simulink model "different_inverter_controls_BPS"  (R2024b)
settings: Solver=ode4  StartTime=0.0  StopTime=5  FixedStep=Ts  RelTol=1e-3
InitFcn:
  | %mode_of_operation=1;
  | %BESS_control_mode=1;
  | %Gen_Q_Control =1;
  | 
  | %Exciter_init;
  | 
  | %Exciter_init
  | Xq=0.474;
  | %%====================================================
  | % ST6C Exciter Parameters
  | 
  | KPA=30;
  | KIA=59.91;
  | KFF=1;
  | KM=1;
  | KLR=22.47;
  | KCL=1.04;
  | VAMAX=7.05;
  | VAMIN=-6.11;
  | VRMAX=7.05;
  | VRMIN=-6.11;
  | ILR=5.02;
  | KG=1;
  | TG=0.024;
  | TA=0.01;
  | VBMAX=999;
  | VMMAX=7.05;
  | VMMIN=-6.11;
  | KI=0;
  | Kp=1;
  | Kc=0;
  | Vt0=0;
  | VAAMAX=VAMAX;
  | %%========================================================
  | % UEL2C parameters
  | 
  | TUQ=.005;
  | TUP=0.050;
  | TUV=0.2;
  | TQREF=0;
  | Tadj=0;
  | K1=0;
  | K2=2;
  | VBIAS=1;
  | KFB=0;
  | TUL=0;
  | VUImax=1;
  | VUImin=-1;
  | VUELmax1=1;
  | VUELmax2=1;
  | VUELmin1=-1;
  | VUELmin2=-1;
  | KUF=0;
  | KUL=0.24;
  | KUI=0.001;
  | TU1=0;TU2=0;TU3=0;TU4=0;
  | KFIX=1;
  | VF=0;
  | VFB=0;
  | %%===========================================================
  | ... (+60 lines)
values from neighbouring files (symbols this model uses):
  inv1 = struct    [multiInverterParams.m]
  kp_sync = KQ_p/10    (= 0.04)    [multiInverterParams.m]
  Vdc = 1000    [multiInverterParams.m]
  Vpp = 480    [multiInverterParams.m]
undefined symbols (not defined in the file or in its folder): D1, Delta, DiscIntNeverNeededParam, Ion, Lithium, sigbuilder_block, sps
libraries: slpidlib x34, spsThreePhaseVIMeasurementLib x31, spsThreePhaseSeriesRLCBranchLib x23, spsabctodq0Lib x22, spsPower3phInstantaneousLib x22, spsThreePhaseTransformerTwoWindingsLib x16, spsSeriesRLCBranchLib x16, spsThreePhaseSeriesRLCLoadLib x14, simulink x12, spsPLL3phLib x11, spsGroundLib x9, powerlib_extras x8
(part 3 of 9)

== system different_inverter_controls_BPS/IBR-GFM Synchro-inverter/Inverter/Grid Inverter ==
  note: Harmonic Filter
  Uref : Inport
  10 kvar1 : spsThreePhaseSeriesRLCLoadLib/Three-Phase Series RLC Load  Commented=on  LConnTagsString=A|B|C  Configuration=Delta  NominalVoltage=Vpp  Vabc=[1e3 1e3 1e3]  Vabcp=[1e3 1e3 1e3]  NominalFrequency=f  UnbalancedPower=off  ActivePower=Pc  InductivePower=0  CapacitivePower=Qc  Pabc=[10e3 9e3 11e3]  QLabc=[100 90 110]  QCabc=[100 90 110]  Pabcp=[10e3 9e3 11e3]  QLabcp=[100 90 110]  QCabcp=[100 90 110]  Measurements=None  LoadType=constant Z
  10 kvar2 : spsThreePhaseSeriesRLCLoadLib/Three-Phase Series RLC Load  Commented=on  LConnTagsString=A|B|C  Configuration=Delta  NominalVoltage=Vpp  Vabc=[1e3 1e3 1e3]  Vabcp=[1e3 1e3 1e3]  NominalFrequency=f  UnbalancedPower=off  ActivePower=Pc  InductivePower=0  CapacitivePower=Qc  Pabc=[10e3 9e3 11e3]  QLabc=[100 90 110]  QCabc=[100 90 110]  Pabcp=[10e3 9e3 11e3]  QLabcp=[100 90 110]  QCabcp=[100 90 110]  Measurements=None  LoadType=constant Z
  B1 : spsThreePhaseVIMeasurementLib/Three-Phase V-I Measurement  VoltageMeasurement=phase-to-ground  SetLabelV=off  LabelV=Vabc_B1  Vpu=off  VpuLL=off  CurrentMeasurement=yes  SetLabelI=off  LabelI=Iabc_B1  Ipu=off  Pbase=100e6  Vbase=500e3  OutputType=Magnitude  PhasorSimulation=off  PSBequivalent=0
  B2 : spsThreePhaseVIMeasurementLib/Three-Phase V-I Measurement  Commented=on  VoltageMeasurement=no  SetLabelV=off  LabelV=Vabc_B1  Vpu=off  VpuLL=off  CurrentMeasurement=yes  SetLabelI=off  LabelI=Iabc_B1  Ipu=on  Pbase=50e6  Vbase=Vnom_sec  OutputType=Magnitude  PhasorSimulation=off  PSBequivalent=0
  B3 : spsThreePhaseVIMeasurementLib/Three-Phase V-I Measurement  VoltageMeasurement=phase-to-ground  SetLabelV=on  LabelV=Vinv  Vpu=on  VpuLL=off  CurrentMeasurement=yes  SetLabelI=on  LabelI=Iinv  Ipu=on  Pbase=110e6  Vbase=Vpp  OutputType=Magnitude  PhasorSimulation=off  PSBequivalent=0
  B4 : spsThreePhaseVIMeasurementLib/Three-Phase V-I Measurement  Commented=on  VoltageMeasurement=phase-to-ground  SetLabelV=on  LabelV=Vinv  Vpu=on  VpuLL=off  CurrentMeasurement=yes  SetLabelI=on  LabelI=Igrid  Ipu=on  Pbase=55e6  Vbase=Vpp  OutputType=Magnitude  PhasorSimulation=off  PSBequivalent=0
  Bus Creator : BusCreator  Inputs=2
  Cf : spsThreePhaseSeriesRLCBranchLib/Three-Phase Series RLC Branch  LConnTagsString=A|B|C  RConnTagsString=A|B|C  BranchType=RC  Resistance=inv1.Rf  Inductance=inv1.L  Capacitance=inv1.Cf  Measurements=None
  Ground : Ground
  Ground1 : spsGroundLib/Ground  LConnTagsString=a
  L1 : spsThreePhaseSeriesRLCBranchLib/Three-Phase Series RLC Branch  LConnTagsString=A|B|C  RConnTagsString=A|B|C  BranchType=RL  Resistance=Rchoke*Zbase  Inductance=inv1.L  Capacitance=inf  Measurements=None
  L2 : spsThreePhaseSeriesRLCBranchLib/Three-Phase Series RLC Branch  Commented=on  LConnTagsString=A|B|C  RConnTagsString=A|B|C  BranchType=RL  Resistance=Rchoke*Zbase  Inductance=Lchoke*Zbase/(2*pi*Fnom)  Capacitance=inf  Measurements=None
  L3 : spsThreePhaseSeriesRLCBranchLib/Three-Phase Series RLC Branch  Commented=on  LConnTagsString=A|B|C  RConnTagsString=A|B|C  BranchType=RL  Resistance=inv1.R  Inductance=inv1.L  Capacitance=inf  Measurements=None
  "Power (3ph, Instantaneous)" : spsPower3phInstantaneousLib/Power (3ph, Instantaneous)
  Scope : Scope  NumInputPorts=2
  Scope1 : Scope  NumInputPorts=2
  Scope2 : Scope
  Three-Level NPC Converter : spsThreeLevelNPCConverterLib/Three-Level NPC Converter  ModelType=Average model (Uref-controlled)  Ron=1e-3  Rs=1e6  Cs=inf  Vforward=[0,0]  Ron_Diode=1e-3  Rs_Diode=1e6  Cs_Diode=inf  Vf_Diode=1e-3  Rs_CurrentSource=inf  Ron_ACsource=1e-3
  XFR : spsThreePhaseTransformerTwoWindingsLib/Three-Phase Transformer (Two Windings)  Winding1Connection=Yg  Winding2Connection=Yg  CoreType=Three single-phase transformers  SetSaturation=off  Hysteresis=off  DataFile='hysteresis'  SetInitialFlux=off  Measurements=None  UNITS=pu  NominalPower=[200e6, f ]  Winding1="[Vpp,  1e-6, 0.0586  ]"  Winding2="[ Vnom_prim,  1e-6, 0.0586  ]"  Rm=500  Lm=500  L0=0.5  Saturation=[ 0,0 ; 0.0024,1.2 ; 1.0,1.52 ]  InitialFluxes=[ 0.8 , -0.8 , 0.7 ]  BreakLoop=off  DiscreteSolver=Trapezoidal iterative  DataType=off  TransfoNumber=1
  XFR1 : spsThreePhaseTransformerTwoWindingsLib/Three-Phase Transformer (Two Windings)  Commented=on  Winding1Connection=Delta (D1)  Winding2Connection=Delta (D1)  CoreType=Three single-phase transformers  SetSaturation=off  Hysteresis=off  DataFile='hysteresis'  SetInitialFlux=off  Measurements=None  UNITS=pu  NominalPower=[100e6, f ]  Winding1="[Vnom_prim,  1e-6, 0.0586 ]"  Winding2="[ Vnom_sec,  1e-6, 0.0586 ]"  Rm=500  Lm=500  L0=0.5  Saturation=[ 0,0 ; 0.0024,1.2 ; 1.0,1.52 ]  InitialFluxes=[ 0.8 , -0.8 , 0.7 ]  BreakLoop=off  DiscreteSolver=Trapezoidal iterative  DataType=off  TransfoNumber=1
  Inv+ : PMIOPort  Side=Left
  N : PMIOPort  Port=2  Side=Left
  Inv-- : PMIOPort  Port=3  Side=Left
  A : PMIOPort  Port=4  Side=Right
  B : PMIOPort  Port=5  Side=Right
  C : PMIOPort  Port=6  Side=Right
  m : Outport  VectorParamsAs1DForOutWhenUnconnected=off
  tag scope: ICabc=global
  wires:
  "Power (3ph, Instantaneous)"/1 -> Scope2/1
  [Iinv] -> Scope1/2
  [Vinv] -> Scope/2
  Uref/1 -> Three-Level NPC Converter/1
  B1/1 -> Scope/1, "Power (3ph, Instantaneous)"/1, Bus Creator/1  "Vabc"
  B1/2 -> [ICabc], Bus Creator/2, Scope1/1, "Power (3ph, Instantaneous)"/2  "Iabc"
  Bus Creator/1 -> m/1
  Ground/1 -> Three-Level NPC Converter/2
  connections:
  XFR/RConn3 -- C/RConn1
  XFR/RConn2 -- B/RConn1
  XFR/RConn1 -- A/RConn1
  B3/RConn3 -- XFR/LConn3
  B3/RConn2 -- XFR/LConn2
  XFR/LConn1 -- B3/RConn1
  B3/LConn3 -- Cf/LConn3 -- 10 kvar1/LConn3 -- B1/RConn3
  10 kvar1/LConn2 -- B3/LConn2 -- Cf/LConn2 -- B1/RConn2
  B3/LConn1 -- Cf/LConn1 -- 10 kvar1/LConn1 -- B1/RConn1
  B1/LConn3 -- L1/RConn3
  B1/LConn2 -- L1/RConn2
  B1/LConn1 -- L1/RConn1
  Cf/RConn2 -- Cf/RConn3 -- Cf/RConn1 -- Ground1/LConn1
  10 kvar2/LConn1 -- L2/RConn1
  L2/RConn3 -- 10 kvar2/LConn3
  L2/RConn2 -- 10 kvar2/LConn2
  Three-Level NPC Converter/LConn3 -- L1/LConn3
  Three-Level NPC Converter/LConn1 -- L1/LConn1
  Three-Level NPC Converter/LConn2 -- L1/LConn2
  Three-Level NPC Converter/RConn1 -- Inv+/RConn1
  Three-Level NPC Converter/RConn3 -- Inv--/RConn1
  N/RConn1 -- Three-Level NPC Converter/RConn2

== system different_inverter_controls_BPS/IBR-GFM Synchro-inverter/Inverter/Inverter Control ==
  Vabc_prim : Inport  PortDimensions=3
  Iabc_prim : Inport  Port=2  PortDimensions=3
  theta : Inport  Port=3
  Vdref : Inport  Port=4
  V_inv_mag : Inport  Port=5
  " voltage control " : Subsystem
  Conversions : Subsystem
  Current Control : Subsystem  TreatAsAtomicUnit=on
  Demux : Demux  Outputs=2
  From : From  Commented=on  GotoTag=Iabc_B5  TagVisibility=global
  From10 : From  Commented=on  GotoTag=idiqPRefL
  From5 : From  Commented=on  GotoTag=theta  TagVisibility=global
  From7 : From  Commented=on  GotoTag=idiqPRef
  Goto5 : Goto  Commented=on  GotoTag=Vabc_prim
  Overmodulation : spsOvermodulationLib/Overmodulation  Commented=on  OverModType=Flat top
  Scope : Scope  NumInputPorts=2
  Scope1 : Scope
  Scope2 : Scope
  Unit Delay : UnitDelay  SampleTime=Ts_Control  HasFrameUpgradeWarning=on
  current limiter : Subsystem  mask{limMax=clMax, limMin=clMin}
      mask prompts: limMax "Max current limit (pu)"; limMin "Min current limit (pu)"
  Uref : Outport  VectorParamsAs1DForOutWhenUnconnected=off
  tag scope: Vd_meas=global, Vq_meas=global, idiqgrid=global, theta=global
  wires:
  Unit Delay/1 -> Uref/1
  [theta] -> Current Control/1(wt)
  From/1 -> Conversions/3(Iabc_grid)
  Conversions/4(IdIq_grid) -> [idiqgrid]
  V_inv_mag/1 -> current limiter/2(V_inv_mag)
  [IdIqref] -> Current Control/4(IdIq_ref)
  [IdIqref] -> current limiter/1(idiqPref)
  Vdref/1 -> " voltage control "/3(Vdref)
  current limiter/1(idiqPRefL) -> [idiqPRefL], Scope/1
  [idiqPRef] -> Scope/2
  Demux/2 -> [Vq_meas]
  Demux/1 -> [Vd_meas]
  [Vd_meas] -> " voltage control "/1(Vd_meas)
  theta/1 -> [theta]
  Conversions/1(wt) -> [wt_GFL]
  Vabc_prim/1 -> Goto5/1, Conversions/1(Vabc_prim)
  [idiqPRef] -> Current Control/3(IdIq_meas)
  Conversions/3(IdIq_prim) -> [idiqPRef]
  Current Control/1(Uabc) -> Unit Delay/1
  Conversions/2(VdVq_prim) -> Demux/1, Scope1/1, Current Control/2(VdVq_meas)
  Iabc_prim/1 -> Conversions/2(Iabc_prim)
  [Vq_meas] -> " voltage control "/2(Vq)
  " voltage control "/1(IdIq_ref.) -> [IdIqref], Scope2/1

== system different_inverter_controls_BPS/IBR-GFM Synchro-inverter/Inverter/Measures ==
  Grid : Inport
  Battery : Inport  Port=2
  Bus Creator : BusCreator  Inputs=2
  Bus Creator1 : BusCreator  Inputs=4
  Bus Selector2 : BusSelector  OutputSignals=Vabc,Iabc
  "Power (3ph, Instantaneous)" : spsPower3phInstantaneousLib/Power (3ph, Instantaneous)
  Scope : Scope
  m : Outport  VectorParamsAs1DForOutWhenUnconnected=off
  wires:
  Bus Creator1/1 -> Bus Creator/1  "Grid"
  "Power (3ph, Instantaneous)"/2 -> Bus Creator1/4  "Q"
  Grid/1 -> Bus Selector2/1
  Battery/1 -> Bus Creator/2  "Battery"
  Bus Creator/1 -> m/1
  "Power (3ph, Instantaneous)"/1 -> Scope/1, Bus Creator1/3  "P"
  Bus Selector2/2 -> Bus Creator1/2, "Power (3ph, Instantaneous)"/2  "<Iabc>"
  Bus Selector2/1 -> Bus Creator1/1, "Power (3ph, Instantaneous)"/1  "<Vabc>"

== system different_inverter_controls_BPS/IBR-GFM Synchro-inverter/Inverter/Power Controller ==
  m_PQ : Inport
  PQref_f : Inport  Port=2
  Input : Inport  Port=3
  fsys : Inport  Port=4
  V_inv_mag : Inport  Port=5
  Compute PQ : Subsystem
  "P,Q Control " : Subsystem  TreatAsAtomicUnit=on
  Scope : Scope
  Scope1 : Scope
  to PU : Gain  Gain=1/Pnom
  theta : Outport  VectorParamsAs1DForOutWhenUnconnected=off
  Vdref : Outport  Port=2
  wires:
  V_inv_mag/1 -> "P,Q Control "/5(V_inv_mag)
  "P,Q Control "/2(Vdref) -> Vdref/1
  "P,Q Control "/1(theta) -> Scope/1, theta/1
  Compute PQ/1(PQm) -> "P,Q Control "/2(m)
  to PU/1 -> "P,Q Control "/1(PQref), Scope1/1
  m_PQ/1 -> Compute PQ/1(m)
  PQref_f/1 -> to PU/1
  Input/1 -> "P,Q Control "/3(w0)
  fsys/1 -> "P,Q Control "/4(fsys)

== system different_inverter_controls_BPS/IBR-GFM Power Synchronization/Inverter/ Reference  ==
  Constant2 : Constant  Value=110e6*.9  SampleTime=Ts_Control
  Constant3 : Constant  Commented=on  Value=55e6*.9  SampleTime=Ts_Control
  Mux3 : Mux  Inputs=2
  Qref : Subsystem
  Scope : Scope
  tag scope: BESS_PQf_ref=global
  wires:
  Constant2/1 -> Mux3/1
  Qref/1(Out1) -> Mux3/2
  Mux3/1 -> [BESS_PQf_ref], Scope/1

== system different_inverter_controls_BPS/IBR-GFM Power Synchronization/Inverter/DC Link ==
  C1 : spsSeriesRLCBranchLib/Series RLC Branch  LConnTagsString=__new0  RConnTagsString=__new0  BranchType=RC  Resistance=10e-5  Inductance=1.0  SetiL0=off  InitialCurrent=0  Capacitance=inv1.C/2  Setx0=on  InitialVoltage=Vdc/2  Measurements=None
  C2 : spsSeriesRLCBranchLib/Series RLC Branch  LConnTagsString=__new0  RConnTagsString=__new0  BranchType=RC  Resistance=10e-5  Inductance=1.0  SetiL0=off  InitialCurrent=0  Capacitance=inv1.C/2  Setx0=on  InitialVoltage=Vdc/2  Measurements=None
  C3 : spsSeriesRLCBranchLib/Series RLC Branch  Commented=on  LConnTagsString=__new0  RConnTagsString=__new0  BranchType=RC  Resistance=10e-5  Inductance=1.0  SetiL0=off  InitialCurrent=0  Capacitance=Clink  Setx0=on  InitialVoltage=Vnom_dc/2  Measurements=None
  PV+ : PMIOPort  Side=Left
  PV-- : PMIOPort  Port=2  Side=Left
  Inv+ : PMIOPort  Port=3  Side=Right
  N : PMIOPort  Port=4  Side=Right
  Inv-- : PMIOPort  Port=5  Side=Right
  connections:
  Inv--/RConn1 -- PV--/RConn1 -- C2/RConn1
  C1/RConn1 -- N/RConn1 -- C2/LConn1
  Inv+/RConn1 -- PV+/RConn1 -- C1/LConn1

== system different_inverter_controls_BPS/IBR-GFM Power Synchronization/Inverter/Grid Inverter ==
  note: Harmonic Filter
  Uref : Inport
  10 kvar1 : spsThreePhaseSeriesRLCLoadLib/Three-Phase Series RLC Load  Commented=on  LConnTagsString=A|B|C  Configuration=Delta  NominalVoltage=Vpp  Vabc=[1e3 1e3 1e3]  Vabcp=[1e3 1e3 1e3]  NominalFrequency=f  UnbalancedPower=off  ActivePower=Pc  InductivePower=0  CapacitivePower=Qc  Pabc=[10e3 9e3 11e3]  QLabc=[100 90 110]  QCabc=[100 90 110]  Pabcp=[10e3 9e3 11e3]  QLabcp=[100 90 110]  QCabcp=[100 90 110]  Measurements=None  LoadType=constant Z
  10 kvar2 : spsThreePhaseSeriesRLCLoadLib/Three-Phase Series RLC Load  Commented=on  LConnTagsString=A|B|C  Configuration=Delta  NominalVoltage=Vpp  Vabc=[1e3 1e3 1e3]  Vabcp=[1e3 1e3 1e3]  NominalFrequency=f  UnbalancedPower=off  ActivePower=Pc  InductivePower=0  CapacitivePower=Qc  Pabc=[10e3 9e3 11e3]  QLabc=[100 90 110]  QCabc=[100 90 110]  Pabcp=[10e3 9e3 11e3]  QLabcp=[100 90 110]  QCabcp=[100 90 110]  Measurements=None  LoadType=constant Z
  B1 : spsThreePhaseVIMeasurementLib/Three-Phase V-I Measurement  VoltageMeasurement=phase-to-ground  SetLabelV=off  LabelV=Vabc_B1  Vpu=off  VpuLL=off  CurrentMeasurement=yes  SetLabelI=off  LabelI=Iabc_B1  Ipu=off  Pbase=100e6  Vbase=500e3  OutputType=Magnitude  PhasorSimulation=off  PSBequivalent=0
  B2 : spsThreePhaseVIMeasurementLib/Three-Phase V-I Measurement  Commented=on  VoltageMeasurement=no  SetLabelV=off  LabelV=Vabc_B1  Vpu=off  VpuLL=off  CurrentMeasurement=yes  SetLabelI=off  LabelI=Iabc_B1  Ipu=on  Pbase=50e6  Vbase=Vnom_sec  OutputType=Magnitude  PhasorSimulation=off  PSBequivalent=0
  B3 : spsThreePhaseVIMeasurementLib/Three-Phase V-I Measurement  VoltageMeasurement=phase-to-ground  SetLabelV=on  LabelV=Vinv  Vpu=on  VpuLL=off  CurrentMeasurement=yes  SetLabelI=on  LabelI=Iinv  Ipu=on  Pbase=110e6  Vbase=Vpp  OutputType=Magnitude  PhasorSimulation=off  PSBequivalent=0
  B4 : spsThreePhaseVIMeasurementLib/Three-Phase V-I Measurement  Commented=on  VoltageMeasurement=phase-to-ground  SetLabelV=on  LabelV=Vinv  Vpu=on  VpuLL=off  CurrentMeasurement=yes  SetLabelI=on  LabelI=Igrid  Ipu=on  Pbase=55e6  Vbase=Vpp  OutputType=Magnitude  PhasorSimulation=off  PSBequivalent=0
  Bus Creator : BusCreator  Inputs=2
  Cf : spsThreePhaseSeriesRLCBranchLib/Three-Phase Series RLC Branch  LConnTagsString=A|B|C  RConnTagsString=A|B|C  BranchType=RC  Resistance=inv1.Rf  Inductance=inv1.L  Capacitance=inv1.Cf  Measurements=None
  Ground : Ground
  Ground1 : spsGroundLib/Ground  LConnTagsString=a
  L1 : spsThreePhaseSeriesRLCBranchLib/Three-Phase Series RLC Branch  LConnTagsString=A|B|C  RConnTagsString=A|B|C  BranchType=RL  Resistance=Rchoke*Zbase  Inductance=inv1.L  Capacitance=inf  Measurements=None
  L2 : spsThreePhaseSeriesRLCBranchLib/Three-Phase Series RLC Branch  Commented=on  LConnTagsString=A|B|C  RConnTagsString=A|B|C  BranchType=RL  Resistance=Rchoke*Zbase  Inductance=Lchoke*Zbase/(2*pi*Fnom)  Capacitance=inf  Measurements=None
  L3 : spsThreePhaseSeriesRLCBranchLib/Three-Phase Series RLC Branch  Commented=on  LConnTagsString=A|B|C  RConnTagsString=A|B|C  BranchType=RL  Resistance=inv1.R  Inductance=inv1.L  Capacitance=inf  Measurements=None
  "Power (3ph, Instantaneous)" : spsPower3phInstantaneousLib/Power (3ph, Instantaneous)
  Scope : Scope  NumInputPorts=2
  Scope1 : Scope  NumInputPorts=2
  Scope2 : Scope
  Three-Level NPC Converter : spsThreeLevelNPCConverterLib/Three-Level NPC Converter  ModelType=Average model (Uref-controlled)  Ron=1e-3  Rs=1e6  Cs=inf  Vforward=[0,0]  Ron_Diode=1e-3  Rs_Diode=1e6  Cs_Diode=inf  Vf_Diode=1e-3  Rs_CurrentSource=inf  Ron_ACsource=1e-3
  XFR : spsThreePhaseTransformerTwoWindingsLib/Three-Phase Transformer (Two Windings)  Winding1Connection=Yg  Winding2Connection=Yg  CoreType=Three single-phase transformers  SetSaturation=off  Hysteresis=off  DataFile='hysteresis'  SetInitialFlux=off  Measurements=None  UNITS=pu  NominalPower=[200e6, f ]  Winding1="[Vpp,  1e-6, 0.0586  ]"  Winding2="[ Vnom_prim,  1e-6, 0.0586  ]"  Rm=500  Lm=500  L0=0.5  Saturation=[ 0,0 ; 0.0024,1.2 ; 1.0,1.52 ]  InitialFluxes=[ 0.8 , -0.8 , 0.7 ]  BreakLoop=off  DiscreteSolver=Trapezoidal iterative  DataType=off  TransfoNumber=1
  XFR1 : spsThreePhaseTransformerTwoWindingsLib/Three-Phase Transformer (Two Windings)  Commented=on  Winding1Connection=Delta (D1)  Winding2Connection=Delta (D1)  CoreType=Three single-phase transformers  SetSaturation=off  Hysteresis=off  DataFile='hysteresis'  SetInitialFlux=off  Measurements=None  UNITS=pu  NominalPower=[100e6, f ]  Winding1="[Vnom_prim,  1e-6, 0.0586 ]"  Winding2="[ Vnom_sec,  1e-6, 0.0586 ]"  Rm=500  Lm=500  L0=0.5  Saturation=[ 0,0 ; 0.0024,1.2 ; 1.0,1.52 ]  InitialFluxes=[ 0.8 , -0.8 , 0.7 ]  BreakLoop=off  DiscreteSolver=Trapezoidal iterative  DataType=off  TransfoNumber=1
  Inv+ : PMIOPort  Side=Left
  N : PMIOPort  Port=2  Side=Left
  Inv-- : PMIOPort  Port=3  Side=Left
  A : PMIOPort  Port=4  Side=Right
  B : PMIOPort  Port=5  Side=Right
  C : PMIOPort  Port=6  Side=Right
  m : Outport  VectorParamsAs1DForOutWhenUnconnected=off
  tag scope: ICabc=global
  wires:
  "Power (3ph, Instantaneous)"/1 -> Scope2/1
  [Iinv] -> Scope1/2
  [Vinv] -> Scope/2
  Uref/1 -> Three-Level NPC Converter/1
  B1/1 -> Scope/1, "Power (3ph, Instantaneous)"/1, Bus Creator/1  "Vabc"
  B1/2 -> [ICabc], Bus Creator/2, Scope1/1, "Power (3ph, Instantaneous)"/2  "Iabc"
  Bus Creator/1 -> m/1
  Ground/1 -> Three-Level NPC Converter/2
  connections:
  XFR/RConn3 -- C/RConn1
  XFR/RConn2 -- B/RConn1
  XFR/RConn1 -- A/RConn1
  B3/RConn3 -- XFR/LConn3
  B3/RConn2 -- XFR/LConn2
  XFR/LConn1 -- B3/RConn1
  B3/LConn3 -- Cf/LConn3 -- 10 kvar1/LConn3 -- B1/RConn3
  10 kvar1/LConn2 -- B3/LConn2 -- Cf/LConn2 -- B1/RConn2
  B3/LConn1 -- Cf/LConn1 -- 10 kvar1/LConn1 -- B1/RConn1
  B1/LConn3 -- L1/RConn3
  B1/LConn2 -- L1/RConn2
  B1/LConn1 -- L1/RConn1
  Cf/RConn2 -- Cf/RConn3 -- Cf/RConn1 -- Ground1/LConn1
  10 kvar2/LConn1 -- L2/RConn1
  L2/RConn3 -- 10 kvar2/LConn3
  L2/RConn2 -- 10 kvar2/LConn2
  Three-Level NPC Converter/LConn3 -- L1/LConn3
  Three-Level NPC Converter/LConn1 -- L1/LConn1
  Three-Level NPC Converter/LConn2 -- L1/LConn2
  Three-Level NPC Converter/RConn1 -- Inv+/RConn1
  Three-Level NPC Converter/RConn3 -- Inv--/RConn1
  N/RConn1 -- Three-Level NPC Converter/RConn2

== system different_inverter_controls_BPS/IBR-GFM Power Synchronization/Inverter/Inverter Control ==
  Vabc_prim : Inport  PortDimensions=3
  Iabc_prim : Inport  Port=2  PortDimensions=3
  theta : Inport  Port=3
  Vdref : Inport  Port=4
  V_inv_mag : Inport  Port=5
  " voltage control " : Subsystem
  Conversions : Subsystem
  Current Control : Subsystem  TreatAsAtomicUnit=on
  Demux : Demux  Outputs=2
  From : From  Commented=on  GotoTag=Iabc_B5  TagVisibility=global
  From10 : From  Commented=on  GotoTag=idiqPRefL
  From5 : From  Commented=on  GotoTag=theta  TagVisibility=global
  From7 : From  Commented=on  GotoTag=idiqPRef
  Goto5 : Goto  Commented=on  GotoTag=Vabc_prim
  Overmodulation : spsOvermodulationLib/Overmodulation  Commented=on  OverModType=Flat top
  Scope : Scope  NumInputPorts=2
  Scope1 : Scope
  Scope2 : Scope
  Unit Delay : UnitDelay  SampleTime=Ts_Control  HasFrameUpgradeWarning=on
  current limiter : Subsystem  mask{limMax=clMax, limMin=clMin}
      mask prompts: limMax "Max current limit (pu)"; limMin "Min current limit (pu)"
  Uref : Outport  VectorParamsAs1DForOutWhenUnconnected=off
  tag scope: Vd_meas=global, Vq_meas=global, idiqgrid=global, theta=global
  wires:
  Unit Delay/1 -> Uref/1
  [theta] -> Current Control/1(wt)
  From/1 -> Conversions/3(Iabc_grid)
  Conversions/4(IdIq_grid) -> [idiqgrid]
  V_inv_mag/1 -> current limiter/2(V_inv_mag)
  [IdIqref] -> Current Control/4(IdIq_ref)
  [IdIqref] -> current limiter/1(idiqPref)
  Vdref/1 -> " voltage control "/3(Vdref)
  current limiter/1(idiqPRefL) -> [idiqPRefL], Scope/1
  [idiqPRef] -> Scope/2
  Demux/2 -> [Vq_meas]
  Demux/1 -> [Vd_meas]
  [Vd_meas] -> " voltage control "/1(Vd_meas)
  theta/1 -> [theta]
  Conversions/1(wt) -> [wt_GFL]
  Vabc_prim/1 -> Goto5/1, Conversions/1(Vabc_prim)
  [idiqPRef] -> Current Control/3(IdIq_meas)
  Conversions/3(IdIq_prim) -> [idiqPRef]
  Current Control/1(Uabc) -> Unit Delay/1
  Conversions/2(VdVq_prim) -> Demux/1, Scope1/1, Current Control/2(VdVq_meas)
  Iabc_prim/1 -> Conversions/2(Iabc_prim)
  [Vq_meas] -> " voltage control "/2(Vq)
  " voltage control "/1(IdIq_ref.) -> [IdIqref], Scope2/1

== system different_inverter_controls_BPS/IBR-GFM Power Synchronization/Inverter/Measures ==
  Grid : Inport
  Battery : Inport  Port=2
  Bus Creator : BusCreator  Inputs=2
  Bus Creator1 : BusCreator  Inputs=4
  Bus Selector2 : BusSelector  OutputSignals=Vabc,Iabc
  "Power (3ph, Instantaneous)" : spsPower3phInstantaneousLib/Power (3ph, Instantaneous)
  Scope : Scope
  m : Outport  VectorParamsAs1DForOutWhenUnconnected=off
  wires:
  Bus Creator1/1 -> Bus Creator/1  "Grid"
  "Power (3ph, Instantaneous)"/2 -> Bus Creator1/4  "Q"
  Grid/1 -> Bus Selector2/1
  Battery/1 -> Bus Creator/2  "Battery"
  Bus Creator/1 -> m/1
  "Power (3ph, Instantaneous)"/1 -> Scope/1, Bus Creator1/3  "P"
  Bus Selector2/2 -> Bus Creator1/2, "Power (3ph, Instantaneous)"/2  "<Iabc>"
  Bus Selector2/1 -> Bus Creator1/1, "Power (3ph, Instantaneous)"/1  "<Vabc>"

== system different_inverter_controls_BPS/IBR-GFM Power Synchronization/Inverter/Power Controller ==
  m_PQ : Inport
  PQref_f : Inport  Port=2
  Input : Inport  Port=3
  fsys : Inport  Port=4
  V_inv_mag : Inport  Port=5
  -180 < alpha < 180 : spsPMUPLLBasedPositiveSequenceLib/PMU (PLL-Based, Positive-Sequence)/-180 < alpha < 180  Commented=on  SystemSampleTime=-1  VariantActivationTime=update diagram  AllowFlexibleInterface=on  Latency=0  AutoFrameSizeCalculation=off
  Compute PQ : Subsystem
  Goto4 : Goto  Commented=on  GotoTag=theta_inv  TagVisibility=global
  "P,Q Control " : Subsystem  TreatAsAtomicUnit=on
  Scope : Scope
  Scope1 : Scope
  to PU : Gain  Gain=1/Pnom
  theta : Outport  VectorParamsAs1DForOutWhenUnconnected=off
  Vdref : Outport  Port=2
  wires:
  V_inv_mag/1 -> "P,Q Control "/5(V_inv_mag)
  "P,Q Control "/2(Vdref) -> Vdref/1
  "P,Q Control "/1(theta) -> Scope/1, Goto4/1, theta/1
  Compute PQ/1(PQm) -> "P,Q Control "/2(m)
  to PU/1 -> "P,Q Control "/1(PQref), Scope1/1
  m_PQ/1 -> Compute PQ/1(m)
  PQref_f/1 -> to PU/1
  Input/1 -> "P,Q Control "/3(w0)
  fsys/1 -> "P,Q Control "/4(fsys)

== system different_inverter_controls_BPS/GFM-VSG-100MW/FRT/In -RSY/3 ph RMS ==
  In1 : Inport
  Add1 : Sum  Inputs=+-
  Add2 : Sum  Inputs=+-
  Add3 : Sum  Inputs=+-
  Add4 : Sum  Inputs=+++
  Demux1 : Demux  Outputs=3
  Math Function : Math  Operator=square
  Math Function1 : Math  Operator=square
  Math Function2 : Math  Operator=square
  RMS2 : spsRMSLib/RMS  TrueRMS=on  Freq=60  RMSInit=1.5  Ts=0
  avg : Gain  Gain=1/3
  avg1 : Gain  Gain=2/3
  Out1 : Outport
  wires:
  Demux1/3 -> Add3/1, Add2/2
  Add3/1 -> Math Function2/1
  Math Function2/1 -> Add4/3
  Demux1/2 -> Add2/1, Add1/2
  In1/1 -> Demux1/1
  avg/1 -> RMS2/1
  Add1/1 -> Math Function/1
  Demux1/1 -> Add3/2, Add1/1
  Math Function1/1 -> Add4/2
  Add4/1 -> avg/1
  Math Function/1 -> Add4/1
  Add2/1 -> Math Function1/1
  RMS2/1 -> avg1/1
  avg1/1 -> Out1/1

== system different_inverter_controls_BPS/GFM-VSG-100MW/FRT/In -RSY/3 ph RMS1 ==
  In1 : Inport
  Add1 : Sum  Inputs=+-
  Add2 : Sum  Inputs=+-
  Add3 : Sum  Inputs=+-
  Add4 : Sum  Inputs=+++
  Demux1 : Demux  Outputs=3
  Math Function : Math  Operator=square
  Math Function1 : Math  Operator=square
  Math Function2 : Math  Operator=square
  RMS2 : spsRMSLib/RMS  TrueRMS=on  Freq=60  RMSInit=1.5  Ts=0
  avg : Gain  Gain=1/3
  avg1 : Gain  Gain=2/3
  Out1 : Outport
  wires:
  Demux1/3 -> Add3/1, Add2/2
  Add3/1 -> Math Function2/1
  Math Function2/1 -> Add4/3
  Demux1/2 -> Add2/1, Add1/2
  In1/1 -> Demux1/1
  avg/1 -> RMS2/1
  Add1/1 -> Math Function/1
  Demux1/1 -> Add3/2, Add1/1
  Math Function1/1 -> Add4/2
  Add4/1 -> avg/1
  Math Function/1 -> Add4/1
  Add2/1 -> Math Function1/1
  RMS2/1 -> avg1/1
  avg1/1 -> Out1/1

== system different_inverter_controls_BPS/GFM-VSG-100MW/FRT/In -RSY/Anti Aliasing Filters ==
  Vabc : Inport  PortDimensions=3
  Uabc : Inport  Port=2  PortDimensions=3
  2nd-Order Filter : powerlib_extras/Discrete  Control Blocks/Discrete  2nd-Order Filter  FilterType=Lowpass  Fo=Fc  Zeta=0.707  Ts=Ts  Initialize=off  Vac_Init=[0.8 -25 60]  Vdc_Init=-0.4  PlotResponse=off  param1=[1 120 0.1]
  2nd-Order Filter{1..2,8..9} (4 alike) : powerlib_extras/Discrete  Control Blocks/Discrete  2nd-Order Filter  FilterType=Lowpass  Fo=Fc  Zeta=0.707  Ts=Ts  Initialize=off  Vac_Init=[0.8 -25 60]  Vdc_Init=-0.4  PlotResponse=off  param1=[1 5000 0.1]
  2nd-Order Filter7 : powerlib_extras/Discrete  Control Blocks/Discrete  2nd-Order Filter  FilterType=Lowpass  Fo=Fc  Zeta=0.707  Ts=Ts  Initialize=off  Vac_Init=[0.8 -25 60]  Vdc_Init=-0.4  PlotResponse=off  param1=[1 120 0.1]
  Demux : Demux  Outputs=3
      settings: DisplayOption=none
  Demux2 : Demux  Outputs=3
      settings: DisplayOption=none
  Mux : Mux  Inputs=3
  Mux2 : Mux  Inputs=3
  " Vabc" : Outport
  " Uabc" : Outport  Port=2
  wires:
  Demux/2 -> 2nd-Order Filter1/1
  Demux/3 -> 2nd-Order Filter2/1
  2nd-Order Filter2/1 -> Mux/3
  2nd-Order Filter1/1 -> Mux/2
  Mux/1 -> " Vabc"/1
  2nd-Order Filter/1 -> Mux/1
  Vabc/1 -> Demux/1
  Demux/1 -> 2nd-Order Filter/1
  Demux2/1 -> 2nd-Order Filter7/1
  Mux2/1 -> " Uabc"/1
  Demux2/3 -> 2nd-Order Filter9/1
  2nd-Order Filter7/1 -> Mux2/1
  2nd-Order Filter9/1 -> Mux2/3
  2nd-Order Filter8/1 -> Mux2/2
  Demux2/2 -> 2nd-Order Filter8/1
  Uabc/1 -> Demux2/1

== system different_inverter_controls_BPS/GFM-VSG-100MW/FRT/In -RSY/Moving Average ==
  In1 : Inport
  Ground1 : Ground
  Terminator1 : Terminator
  Out1 : Outport
  wires:
  Ground1/1 -> Out1/1
  In1/1 -> Terminator1/1

== system different_inverter_controls_BPS/GFM-VSG-100MW/FRT/In -RSY/PLL0 ==
  note: Discrete time PLL
  vabc : Inport
  2nd-Order Filter : powerlib_extras/Discrete  Control Blocks/Discrete  2nd-Order Filter  FilterType=Lowpass  Fo=25  Zeta=0.707  Ts=Ts_Control  Initialize=off  Vac_Init=[0.8 -25 60]  Vdc_Init=-0.4  PlotResponse=off  param1=[1 120 0.1]
  Constant1 : Constant  Value=0
  Constant2 : Constant
  Constant3 : Constant  Value=2*pi
  Delay2 : Delay  DelayLength=1
  Discrete-Time Integrator : DiscreteIntegrator  ExternalReset=rising  InitialConditionSource=external  SampleTime=Ts_Control  ShowStatePort=on  ICPrevOutput=DiscIntNeverNeededParam  ICPrevScaledInput=DiscIntNeverNeededParam
  Gain1 : Gain  Gain=1/(2*pi)
  Gain2 : Gain  Gain=2*pi*f
  Gain3 : Gain
  GreaterThan : RelationalOperator  Operator=>  OutDataTypeStr=boolean  RndMeth=Simplest  InputSameDT=off
  IC : InitialCondition  Value=0
  Moving Average1 : Subsystem  Description=Replaced Block  Commented=on  InitFcn=error('This block was designed with a newer version of Simulink. Unfortunately, your Simulink version does not support these features.')  mask(Replaced Block){}
      mask help: This block has been replaced with an empty subsystem because it used functionality that is unavailable in Simulink R2021a.
      mask Display: fprintf('Replaced: %s\n','Moving Statistics with Overlap Length not equal to Window Length - 1 (supported from R2022b).')
  PI : Subsystem
  PLL (3ph) : spsPLL3phLib/PLL (3ph)  Commented=on  Fmin=45  Par_Init=[0, 60]  ParK=[180, 3200, 1]  TcD=1e-4  MaxRateChangeFreq=12  FilterCutOffFreq=25  Ts=0  AGC=on
  Scope1 : Scope  NumInputPorts=2
  Selector : Selector  InputPortWidth=3  IndexOptions=Index vector (dialog)  Indices=2  OutputSizes=1
  Subsystem : Subsystem  Commented=on
  Sum : Sum  Inputs=|+-
  Sum2 : Sum  Inputs=|-+
  Sum3 : Sum  Inputs=-+
  abc to dq0 : spsabctodq0Lib/abc to dq0  Alignment=90 degrees behind phase A axis
  fGrid : Outport  VectorParamsAs1DForOutWhenUnconnected=off
  wtGrid : Outport  Port=2  VectorParamsAs1DForOutWhenUnconnected=off
  wires:
  Constant1/1 -> Sum2/2
  Discrete-Time Integrator/State -> GreaterThan/1, Sum/1
  Constant3/1 -> Sum/2, GreaterThan/2
  Sum/1 -> IC/1
  GreaterThan/1 -> Discrete-Time Integrator/2
  IC/1 -> Discrete-Time Integrator/3
  Delay2/1 -> Scope1/2, Sum2/1, Scope1/1
  Gain2/1 -> Discrete-Time Integrator/1, Gain1/1
  PI/1(Out1) -> Gain3/1
  Selector/1 -> Delay2/1  "Vq"
  Sum2/1 -> PI/1(In1)
  Gain1/1 -> 2nd-Order Filter/1
  Constant2/1 -> Sum3/2
  vabc/1 -> abc to dq0/1
  abc to dq0/1 -> Selector/1
  Discrete-Time Integrator/1 -> abc to dq0/2, wtGrid/1
  Gain3/1 -> Sum3/1
  Sum3/1 -> Gain2/1
  2nd-Order Filter/1 -> fGrid/1

== system different_inverter_controls_BPS/GFM-VSG-100MW/FRT/In -RSY/PLL3 ==
  vabc : Inport
  2nd-Order Filter : powerlib_extras/Discrete  Control Blocks/Discrete  2nd-Order Filter  FilterType=Lowpass  Fo=25  Zeta=0.707  Ts=Ts_Control  Initialize=off  Vac_Init=[0.8 -25 60]  Vdc_Init=-0.4  PlotResponse=off  param1=[1 120 0.1]
  Constant1 : Constant  Value=0
  Constant2 : Constant
  Constant3 : Constant  Value=2*pi
  Delay2 : Delay  DelayLength=1
  Discrete-Time Integrator : DiscreteIntegrator  ExternalReset=rising  InitialConditionSource=external  SampleTime=Ts_Control  ShowStatePort=on  ICPrevOutput=DiscIntNeverNeededParam  ICPrevScaledInput=DiscIntNeverNeededParam
  Gain1 : Gain  Gain=1/(2*pi)
  Gain2 : Gain  Gain=2*pi*f
  Gain3 : Gain
  GreaterThan : RelationalOperator  Operator=>  OutDataTypeStr=boolean  RndMeth=Simplest  InputSameDT=off
  IC : InitialCondition  Value=0
  Moving Average1 : Subsystem  Description=Replaced Block  Commented=on  InitFcn=error('This block was designed with a newer version of Simulink. Unfortunately, your Simulink version does not support these features.')  mask(Replaced Block){}
      mask help: This block has been replaced with an empty subsystem because it used functionality that is unavailable in Simulink R2021a.
      mask Display: fprintf('Replaced: %s\n','Moving Statistics with Overlap Length not equal to Window Length - 1 (supported from R2022b).')
  PI : Subsystem
  Scope1 : Scope  NumInputPorts=2
  Selector : Selector  InputPortWidth=3  IndexOptions=Index vector (dialog)  Indices=2  OutputSizes=1
  Subsystem : Subsystem  Commented=on
  Sum : Sum  Inputs=|+-
  Sum2 : Sum  Inputs=|-+
  Sum3 : Sum  Inputs=-+
  abc to dq0 : spsabctodq0Lib/abc to dq0  Alignment=90 degrees behind phase A axis
  fPCC : Outport  VectorParamsAs1DForOutWhenUnconnected=off
  wtPCC : Outport  Port=2  VectorParamsAs1DForOutWhenUnconnected=off
  wires:
  Constant3/1 -> Sum/2, GreaterThan/2
  Sum/1 -> IC/1
  Discrete-Time Integrator/State -> GreaterThan/1, Sum/1
  Constant1/1 -> Sum2/2
  IC/1 -> Discrete-Time Integrator/3
  GreaterThan/1 -> Discrete-Time Integrator/2
  Discrete-Time Integrator/1 -> abc to dq0/2, wtPCC/1
  Gain1/1 -> 2nd-Order Filter/1
  Constant2/1 -> Sum3/2
  Sum3/1 -> Gain2/1
  Gain2/1 -> Discrete-Time Integrator/1, Gain1/1
  Gain3/1 -> Sum3/1
  abc to dq0/1 -> Selector/1
  vabc/1 -> abc to dq0/1
  Selector/1 -> Delay2/1  "Vq"
  Sum2/1 -> PI/1(In1)
  PI/1(Out1) -> Gain3/1
  Delay2/1 -> Scope1/2, Sum2/1, Scope1/1
  2nd-Order Filter/1 -> fPCC/1

== system different_inverter_controls_BPS/GFM-VSG-100MW/FRT/In -RSY/Sync Check Control ==
  In1 : Inport
  PI1 : Subsystem
  SC : Constant  Value=0  SampleTime=Ts_Control
  Switch1 : Switch  Criteria=u2 > Threshold  SaturateOnIntegerOverflow=off  InputSameDT=off
  Trigonometric Function1 : Trigonometry  Commented=on
  Out1 : Outport
  wires:
  SC/1 -> Switch1/3
  PI1/1(Out1) -> Out1/1
  In1/1 -> PI1/1(In1)

== system different_inverter_controls_BPS/GFM-VSG-100MW/FRT/In -RSY/grid health check logic V FRT ==
  In1 : Inport
  Rtot_pu3 : Gain  Gain=100  SaturateOnIntegerOverflow=on  OutDataTypeStr=Inherit: Same as input  ParamDataTypeStr=Inherit: Same as input
  Unit Delay1 : UnitDelay  InitialCondition=1  SampleTime=Ts_Control  HasFrameUpgradeWarning=on
  grid health : MATLAB Function  TreatAsAtomicUnit=on
  t3 : DigitalClock  SampleTime=Ts
  Out1 : Outport
  wires:
  t3/1 -> grid health/2(c)
  Rtot_pu3/1 -> grid health/1(u)
  In1/1 -> Rtot_pu3/1
  grid health/1(y) -> Unit Delay1/1
  Unit Delay1/1 -> Out1/1

== system different_inverter_controls_BPS/GFM-VSG-100MW/FRT/In -RSY/grid health check logic f FRT ==
  In1 : Inport
  Rtot_pu3 : Gain  SaturateOnIntegerOverflow=on  OutDataTypeStr=Inherit: Same as input  ParamDataTypeStr=Inherit: Same as input
  Unit Delay1 : UnitDelay  InitialCondition=1  SampleTime=Ts_Control  HasFrameUpgradeWarning=on
  grid health : MATLAB Function  TreatAsAtomicUnit=on
  t3 : DigitalClock  SampleTime=Ts
  Out1 : Outport
  wires:
  Unit Delay1/1 -> Out1/1
  grid health/1(y) -> Unit Delay1/1
  In1/1 -> Rtot_pu3/1
  Rtot_pu3/1 -> grid health/1(u)
  t3/1 -> grid health/2(c)

== system different_inverter_controls_BPS/GFM-VSG-100MW/FRT/In -RSY/sequence extraction1 ==
  In1 : Inport
  Add1 : Sum
  Add2 : Sum  Inputs=+-
  Add3 : Sum
  Add4 : Sum  Inputs=+-
  Alpha-Beta-Zero to abc : spsAlphaBetaZerotoabcLib/Alpha-Beta-Zero to abc
  Alpha-Beta-Zero to abc1 : spsAlphaBetaZerotoabcLib/Alpha-Beta-Zero to abc
  Delay : Delay  DelayLength=ceil(((1/f)/4)/Ts_Control)
  Delay1 : Delay  DelayLength=ceil(((1/f)/4)/Ts_Control)
  Demux1 : Demux  Outputs=3
  Mux2 : Mux  Inputs=3
  Mux3 : Mux  Inputs=3
  Rtot_pu{1..4} (4 alike) : Gain  Gain=0.5  SaturateOnIntegerOverflow=on  OutDataTypeStr=Inherit: Same as input  ParamDataTypeStr=Inherit: Same as input
  Vdc_ref2 : Constant  Value=0  SampleTime=Ts_Control
  Vdc_ref3 : Constant  Value=0  SampleTime=Ts_Control
  abc to Alpha-Beta-Zero : spsabctoAlphaBetaZeroLib/abc to Alpha-Beta-Zero
  abcP : Outport
  abcN : Outport  Port=2
  wires:
  abc to Alpha-Beta-Zero/1 -> Demux1/1
  In1/1 -> abc to Alpha-Beta-Zero/1
  Alpha-Beta-Zero to abc/1 -> abcP/1
  Vdc_ref2/1 -> Mux2/3
  Alpha-Beta-Zero to abc1/1 -> abcN/1
  Vdc_ref3/1 -> Mux3/3
  Add2/1 -> Rtot_pu3/1
  Add1/1 -> Rtot_pu1/1
  Add3/1 -> Rtot_pu2/1
  Add4/1 -> Rtot_pu4/1
  Rtot_pu3/1 -> Mux2/1
  Rtot_pu4/1 -> Mux3/2
  Demux1/1 -> Delay/1, Add1/1, Add2/1
  Demux1/2 -> Delay1/1, Add3/1, Add4/1
  Delay/1 -> Add4/2, Add3/2
  Delay1/1 -> Add2/2, Add1/2
  Mux2/1 -> Alpha-Beta-Zero to abc/1
  Mux3/1 -> Alpha-Beta-Zero to abc1/1
  Rtot_pu2/1 -> Mux2/2
  Rtot_pu1/1 -> Mux3/1

== system different_inverter_controls_BPS/GFM-VSG-100MW/FRT/In -RSY/sequence extraction4 ==
  In1 : Inport
  Add1 : Sum
  Add2 : Sum  Inputs=+-
  Add3 : Sum
  Add4 : Sum  Inputs=+-
  Alpha-Beta-Zero to abc : spsAlphaBetaZerotoabcLib/Alpha-Beta-Zero to abc
  Alpha-Beta-Zero to abc1 : spsAlphaBetaZerotoabcLib/Alpha-Beta-Zero to abc
  Delay : Delay  DelayLength=ceil(((1/f)/4)/Ts_Control)
  Delay1 : Delay  DelayLength=ceil(((1/f)/4)/Ts_Control)
  Demux1 : Demux  Outputs=3
  Mux2 : Mux  Inputs=3
  Mux3 : Mux  Inputs=3
  Rtot_pu{1..4} (4 alike) : Gain  Gain=0.5  SaturateOnIntegerOverflow=on  OutDataTypeStr=Inherit: Same as input  ParamDataTypeStr=Inherit: Same as input
  Vdc_ref2 : Constant  Value=0  SampleTime=Ts_Control
  Vdc_ref3 : Constant  Value=0  SampleTime=Ts_Control
  abc to Alpha-Beta-Zero : spsabctoAlphaBetaZeroLib/abc to Alpha-Beta-Zero
  abcP : Outport
  abcN : Outport  Port=2
  wires:
  abc to Alpha-Beta-Zero/1 -> Demux1/1
  In1/1 -> abc to Alpha-Beta-Zero/1
  Alpha-Beta-Zero to abc/1 -> abcP/1
  Vdc_ref2/1 -> Mux2/3
  Alpha-Beta-Zero to abc1/1 -> abcN/1
  Vdc_ref3/1 -> Mux3/3
  Add2/1 -> Rtot_pu3/1
  Add1/1 -> Rtot_pu1/1
  Add3/1 -> Rtot_pu2/1
  Add4/1 -> Rtot_pu4/1
  Rtot_pu3/1 -> Mux2/1
  Rtot_pu4/1 -> Mux3/2
  Demux1/1 -> Delay/1, Add1/1, Add2/1
  Demux1/2 -> Delay1/1, Add3/1, Add4/1
  Delay/1 -> Add4/2, Add3/2
  Delay1/1 -> Add2/2, Add1/2
  Mux2/1 -> Alpha-Beta-Zero to abc/1
  Mux3/1 -> Alpha-Beta-Zero to abc1/1
  Rtot_pu2/1 -> Mux2/2
  Rtot_pu1/1 -> Mux3/1

== system different_inverter_controls_BPS/GFM-VSG-100MW/FRT/In -RSY/sync check logic ==
  In1 : Inport
  In2 : Inport  Port=2
  In3 : Inport  Port=3
  Cast To Boolean : DataTypeConversion  OutDataTypeStr=boolean  SaturateOnIntegerOverflow=off  RndMeth=Floor
  Scope8 : Scope  NumInputPorts=3
  Unit Delay1 : UnitDelay  InitialCondition=1  SampleTime=-1  HasFrameUpgradeWarning=on
  sync check : MATLAB Function  TreatAsAtomicUnit=on
  t3 : DigitalClock  SampleTime=Ts
  Out1 : Outport
  wires:
  t3/1 -> sync check/4(tim)
  In1/1 -> Scope8/1, sync check/1(du)
  sync check/1(y) -> Cast To Boolean/1
  Cast To Boolean/1 -> Unit Delay1/1
  In3/1 -> Scope8/3, sync check/3(dth)
  In2/1 -> Scope8/2, sync check/2(df)
  Unit Delay1/1 -> Out1/1

== system different_inverter_controls_BPS/GFM-VSG-100MW/IBR-GFM VSG/Inverter/BESS Reference  ==
  Constant2 : Constant  Value=100e6  SampleTime=Ts_Control
  Mux3 : Mux  Inputs=2
  Qref : Subsystem
  Scope : Scope
  tag scope: BESS_PQf_ref=global
  wires:
  Mux3/1 -> Scope/1, [BESS_PQf_ref]
  Qref/1(Out1) -> Mux3/2
  Constant2/1 -> Mux3/1

== system different_inverter_controls_BPS/GFM-VSG-100MW/IBR-GFM VSG/Inverter/DC Link ==
  C1 : spsSeriesRLCBranchLib/Series RLC Branch  LConnTagsString=__new0  RConnTagsString=__new0  BranchType=RC  Resistance=10e-5  Inductance=1.0  SetiL0=off  InitialCurrent=0  Capacitance=inv1.C/2  Setx0=on  InitialVoltage=Vdc/2  Measurements=None
  C2 : spsSeriesRLCBranchLib/Series RLC Branch  LConnTagsString=__new0  RConnTagsString=__new0  BranchType=RC  Resistance=10e-5  Inductance=1.0  SetiL0=off  InitialCurrent=0  Capacitance=inv1.C/2  Setx0=on  InitialVoltage=Vdc/2  Measurements=None
  C3 : spsSeriesRLCBranchLib/Series RLC Branch  Commented=on  LConnTagsString=__new0  RConnTagsString=__new0  BranchType=RC  Resistance=10e-5  Inductance=1.0  SetiL0=off  InitialCurrent=0  Capacitance=Clink  Setx0=on  InitialVoltage=Vnom_dc/2  Measurements=None
  PV+ : PMIOPort  Side=Left
  PV-- : PMIOPort  Port=2  Side=Left
  Inv+ : PMIOPort  Port=3  Side=Right
  N : PMIOPort  Port=4  Side=Right
  Inv-- : PMIOPort  Port=5  Side=Right
  connections:
  C1/LConn1 -- PV+/RConn1 -- Inv+/RConn1
  C2/LConn1 -- N/RConn1 -- C1/RConn1
  C2/RConn1 -- PV--/RConn1 -- Inv--/RConn1

== system different_inverter_controls_BPS/GFM-VSG-100MW/IBR-GFM VSG/Inverter/Grid Inverter ==
  note: Harmonic Filter
  Uref : Inport
  10 kvar1 : spsThreePhaseSeriesRLCLoadLib/Three-Phase Series RLC Load  Commented=on  LConnTagsString=A|B|C  Configuration=Delta  NominalVoltage=Vpp  Vabc=[1e3 1e3 1e3]  Vabcp=[1e3 1e3 1e3]  NominalFrequency=f  UnbalancedPower=off  ActivePower=Pc  InductivePower=0  CapacitivePower=Qc  Pabc=[10e3 9e3 11e3]  QLabc=[100 90 110]  QCabc=[100 90 110]  Pabcp=[10e3 9e3 11e3]  QLabcp=[100 90 110]  QCabcp=[100 90 110]  Measurements=None  LoadType=constant Z
  10 kvar2 : spsThreePhaseSeriesRLCLoadLib/Three-Phase Series RLC Load  Commented=on  LConnTagsString=A|B|C  Configuration=Delta  NominalVoltage=Vpp  Vabc=[1e3 1e3 1e3]  Vabcp=[1e3 1e3 1e3]  NominalFrequency=f  UnbalancedPower=off  ActivePower=Pc  InductivePower=0  CapacitivePower=Qc  Pabc=[10e3 9e3 11e3]  QLabc=[100 90 110]  QCabc=[100 90 110]  Pabcp=[10e3 9e3 11e3]  QLabcp=[100 90 110]  QCabcp=[100 90 110]  Measurements=None  LoadType=constant Z
  B1 : spsThreePhaseVIMeasurementLib/Three-Phase V-I Measurement  VoltageMeasurement=phase-to-ground  SetLabelV=off  LabelV=Vabc_B1  Vpu=off  VpuLL=off  CurrentMeasurement=yes  SetLabelI=off  LabelI=Iabc_B1  Ipu=off  Pbase=100e6  Vbase=500e3  OutputType=Magnitude  PhasorSimulation=off  PSBequivalent=0
  B2 : spsThreePhaseVIMeasurementLib/Three-Phase V-I Measurement  Commented=on  VoltageMeasurement=no  SetLabelV=off  LabelV=Vabc_B1  Vpu=off  VpuLL=off  CurrentMeasurement=yes  SetLabelI=off  LabelI=Iabc_B1  Ipu=on  Pbase=50e6  Vbase=Vnom_sec  OutputType=Magnitude  PhasorSimulation=off  PSBequivalent=0
  B3 : spsThreePhaseVIMeasurementLib/Three-Phase V-I Measurement  VoltageMeasurement=phase-to-ground  SetLabelV=on  LabelV=Vinv  Vpu=on  VpuLL=off  CurrentMeasurement=yes  SetLabelI=on  LabelI=Iinv  Ipu=on  Pbase=110e6  Vbase=Vpp  OutputType=Magnitude  PhasorSimulation=off  PSBequivalent=0
  B4 : spsThreePhaseVIMeasurementLib/Three-Phase V-I Measurement  Commented=on  VoltageMeasurement=phase-to-ground  SetLabelV=on  LabelV=Vinv  Vpu=on  VpuLL=off  CurrentMeasurement=yes  SetLabelI=on  LabelI=Igrid  Ipu=on  Pbase=55e6  Vbase=Vpp  OutputType=Magnitude  PhasorSimulation=off  PSBequivalent=0
  Bus Creator : BusCreator  Inputs=2
  Cf : spsThreePhaseSeriesRLCBranchLib/Three-Phase Series RLC Branch  LConnTagsString=A|B|C  RConnTagsString=A|B|C  BranchType=RC  Resistance=inv1.Rf  Inductance=inv1.L  Capacitance=inv1.Cf  Measurements=None
  Ground : Ground
  Ground1 : spsGroundLib/Ground  LConnTagsString=a
  L1 : spsThreePhaseSeriesRLCBranchLib/Three-Phase Series RLC Branch  LConnTagsString=A|B|C  RConnTagsString=A|B|C  BranchType=RL  Resistance=Rchoke*Zbase  Inductance=inv1.L  Capacitance=inf  Measurements=None
  L2 : spsThreePhaseSeriesRLCBranchLib/Three-Phase Series RLC Branch  Commented=on  LConnTagsString=A|B|C  RConnTagsString=A|B|C  BranchType=RL  Resistance=Rchoke*Zbase  Inductance=Lchoke*Zbase/(2*pi*Fnom)  Capacitance=inf  Measurements=None
  L3 : spsThreePhaseSeriesRLCBranchLib/Three-Phase Series RLC Branch  Commented=on  LConnTagsString=A|B|C  RConnTagsString=A|B|C  BranchType=RL  Resistance=inv1.R  Inductance=inv1.L  Capacitance=inf  Measurements=None
  "Power (3ph, Instantaneous)" : spsPower3phInstantaneousLib/Power (3ph, Instantaneous)
  Scope : Scope  NumInputPorts=2
  Scope1 : Scope  NumInputPorts=2
  Scope2 : Scope
  Three-Level NPC Converter : spsThreeLevelNPCConverterLib/Three-Level NPC Converter  ModelType=Average model (Uref-controlled)  Ron=1e-3  Rs=1e6  Cs=inf  Vforward=[0,0]  Ron_Diode=1e-3  Rs_Diode=1e6  Cs_Diode=inf  Vf_Diode=1e-3  Rs_CurrentSource=inf  Ron_ACsource=1e-3
  XFR : spsThreePhaseTransformerTwoWindingsLib/Three-Phase Transformer (Two Windings)  Winding1Connection=Yg  Winding2Connection=Yg  CoreType=Three single-phase transformers  SetSaturation=off  Hysteresis=off  DataFile='hysteresis'  SetInitialFlux=off  Measurements=None  UNITS=pu  NominalPower=[200e6, f ]  Winding1="[Vpp,  1e-6, 0.0586  ]"  Winding2="[ Vnom_prim,  1e-6, 0.0586  ]"  Rm=500  Lm=500  L0=0.5  Saturation=[ 0,0 ; 0.0024,1.2 ; 1.0,1.52 ]  InitialFluxes=[ 0.8 , -0.8 , 0.7 ]  BreakLoop=off  DiscreteSolver=Trapezoidal iterative  DataType=off  TransfoNumber=1
  XFR1 : spsThreePhaseTransformerTwoWindingsLib/Three-Phase Transformer (Two Windings)  Commented=on  Winding1Connection=Delta (D1)  Winding2Connection=Delta (D1)  CoreType=Three single-phase transformers  SetSaturation=off  Hysteresis=off  DataFile='hysteresis'  SetInitialFlux=off  Measurements=None  UNITS=pu  NominalPower=[100e6, f ]  Winding1="[Vnom_prim,  1e-6, 0.0586 ]"  Winding2="[ Vnom_sec,  1e-6, 0.0586 ]"  Rm=500  Lm=500  L0=0.5  Saturation=[ 0,0 ; 0.0024,1.2 ; 1.0,1.52 ]  InitialFluxes=[ 0.8 , -0.8 , 0.7 ]  BreakLoop=off  DiscreteSolver=Trapezoidal iterative  DataType=off  TransfoNumber=1
  Inv+ : PMIOPort  Side=Left
  N : PMIOPort  Port=2  Side=Left
  Inv-- : PMIOPort  Port=3  Side=Left
  A : PMIOPort  Port=4  Side=Right
  B : PMIOPort  Port=5  Side=Right
  C : PMIOPort  Port=6  Side=Right
  m : Outport  VectorParamsAs1DForOutWhenUnconnected=off
  tag scope: ICabc=global
  wires:
  Ground/1 -> Three-Level NPC Converter/2
  Bus Creator/1 -> m/1
  B1/2 -> "Power (3ph, Instantaneous)"/2, Scope1/1, Bus Creator/2, [ICabc]  "Iabc"
  B1/1 -> Bus Creator/1, "Power (3ph, Instantaneous)"/1, Scope/1  "Vabc"
  Uref/1 -> Three-Level NPC Converter/1
  [Vinv] -> Scope/2
  [Iinv] -> Scope1/2
  "Power (3ph, Instantaneous)"/1 -> Scope2/1
  connections:
  N/RConn1 -- Three-Level NPC Converter/RConn2
  Three-Level NPC Converter/RConn3 -- Inv--/RConn1
  Three-Level NPC Converter/RConn1 -- Inv+/RConn1
  Three-Level NPC Converter/LConn2 -- L1/LConn2
  Three-Level NPC Converter/LConn1 -- L1/LConn1
  Three-Level NPC Converter/LConn3 -- L1/LConn3
  L2/RConn2 -- 10 kvar2/LConn2
  L2/RConn3 -- 10 kvar2/LConn3
  10 kvar2/LConn1 -- L2/RConn1
  Ground1/LConn1 -- Cf/RConn1 -- Cf/RConn3 -- Cf/RConn2
  B1/LConn1 -- L1/RConn1
  B1/LConn2 -- L1/RConn2
  B1/LConn3 -- L1/RConn3
  B1/RConn1 -- 10 kvar1/LConn1 -- Cf/LConn1 -- B3/LConn1
  B1/RConn2 -- Cf/LConn2 -- B3/LConn2 -- 10 kvar1/LConn2
  B1/RConn3 -- 10 kvar1/LConn3 -- Cf/LConn3 -- B3/LConn3
  XFR/LConn1 -- B3/RConn1
  B3/RConn2 -- XFR/LConn2
  B3/RConn3 -- XFR/LConn3
  XFR/RConn1 -- A/RConn1
  XFR/RConn2 -- B/RConn1
  XFR/RConn3 -- C/RConn1

== system different_inverter_controls_BPS/GFM-VSG-100MW/IBR-GFM VSG/Inverter/Inverter Control ==
  Vabc_prim : Inport  PortDimensions=3
  Iabc_prim : Inport  Port=2  PortDimensions=3
  theta : Inport  Port=3
  Vdref : Inport  Port=4
  V_inv_mag : Inport  Port=5
  " voltage control " : Subsystem
  Conversions : Subsystem
  Current Control : Subsystem  TreatAsAtomicUnit=on
  Demux : Demux  Outputs=2
  From : From  Commented=on  GotoTag=Iabc_B5  TagVisibility=global
  From10 : From  Commented=on  GotoTag=idiqPRefL
  From5 : From  Commented=on  GotoTag=theta  TagVisibility=global
  From7 : From  Commented=on  GotoTag=idiqPRef
  Goto5 : Goto  Commented=on  GotoTag=Vabc_prim
  Overmodulation : spsOvermodulationLib/Overmodulation  Commented=on  OverModType=Flat top
  Scope : Scope  NumInputPorts=2
  Scope1 : Scope
  Scope2 : Scope
  Unit Delay : UnitDelay  SampleTime=Ts_Control  HasFrameUpgradeWarning=on
  current limiter : Subsystem  mask{limMax=clMax, limMin=clMin}
      mask prompts: limMax "Max current limit (pu)"; limMin "Min current limit (pu)"
  Uref : Outport  VectorParamsAs1DForOutWhenUnconnected=off
  tag scope: Vd_meas=global, Vq_meas=global, idiqgrid=global, theta=global
  wires:
  " voltage control "/1(IdIq_ref.) -> Scope2/1, [IdIqref]
  [Vq_meas] -> " voltage control "/2(Vq)
  Iabc_prim/1 -> Conversions/2(Iabc_prim)
  Conversions/2(VdVq_prim) -> Current Control/2(VdVq_meas), Scope1/1, Demux/1
  Current Control/1(Uabc) -> Unit Delay/1
  Conversions/3(IdIq_prim) -> [idiqPRef]
  [idiqPRef] -> Current Control/3(IdIq_meas)
  Vabc_prim/1 -> Conversions/1(Vabc_prim), Goto5/1
  Conversions/1(wt) -> [wt_GFL]
  theta/1 -> [theta]
  [Vd_meas] -> " voltage control "/1(Vd_meas)
  Demux/1 -> [Vd_meas]
  Demux/2 -> [Vq_meas]
  [idiqPRef] -> Scope/2
  current limiter/1(idiqPRefL) -> Scope/1, [idiqPRefL]
  Vdref/1 -> " voltage control "/3(Vdref)
  [IdIqref] -> current limiter/1(idiqPref)
  [IdIqref] -> Current Control/4(IdIq_ref)
  V_inv_mag/1 -> current limiter/2(V_inv_mag)
  Conversions/4(IdIq_grid) -> [idiqgrid]
  From/1 -> Conversions/3(Iabc_grid)
  [theta] -> Current Control/1(wt)
  Unit Delay/1 -> Uref/1

== system different_inverter_controls_BPS/GFM-VSG-100MW/IBR-GFM VSG/Inverter/Measures ==
  Grid : Inport
  Battery : Inport  Port=2
  Bus Creator : BusCreator  Inputs=2
  Bus Creator1 : BusCreator  Inputs=4
  Bus Selector2 : BusSelector  OutputSignals=Vabc,Iabc
  "Power (3ph, Instantaneous)" : spsPower3phInstantaneousLib/Power (3ph, Instantaneous)
  Scope : Scope
  m : Outport  VectorParamsAs1DForOutWhenUnconnected=off
  wires:
  Bus Selector2/1 -> "Power (3ph, Instantaneous)"/1, Bus Creator1/1  "<Vabc>"
  Bus Selector2/2 -> "Power (3ph, Instantaneous)"/2, Bus Creator1/2  "<Iabc>"
  "Power (3ph, Instantaneous)"/1 -> Bus Creator1/3, Scope/1  "P"
  Bus Creator/1 -> m/1
  Battery/1 -> Bus Creator/2  "Battery"
  Grid/1 -> Bus Selector2/1
  "Power (3ph, Instantaneous)"/2 -> Bus Creator1/4  "Q"
  Bus Creator1/1 -> Bus Creator/1  "Grid"

== system different_inverter_controls_BPS/GFM-VSG-100MW/IBR-GFM VSG/Inverter/Power Controller ==
  m_PQ : Inport
  PQref_f : Inport  Port=2
  V_inv_mag : Inport  Port=3
  Compute PQ : Subsystem
  "P,Q Control " : Subsystem  TreatAsAtomicUnit=on
  Scope : Scope
  Scope1 : Scope
  to PU : Gain  Gain=1/Pnom
  theta : Outport  VectorParamsAs1DForOutWhenUnconnected=off
  Vdref : Outport  Port=2
  wires:
  PQref_f/1 -> to PU/1
  m_PQ/1 -> Compute PQ/1(m)
  to PU/1 -> Scope1/1, "P,Q Control "/1(PQref)
  Compute PQ/1(PQm) -> "P,Q Control "/2(m)
  "P,Q Control "/1(theta) -> theta/1, Scope/1
  "P,Q Control "/2(Vdref) -> Vdref/1
  V_inv_mag/1 -> "P,Q Control "/3(V_inv_mag)
